simulink model "ServerExpCM_Model"  (R2023a)
settings: Solver=VariableStepAuto  StartTime=0.0  StopTime=10.0  RelTol=1e-3
libraries: NSA_DEVS_SINKS_ATOMIC x5, TimeSharedLib x4, NSA_DEVS_LOGISTICS_ATOMIC x2, NSA_DEVS_SOURCES_ATOMIC x1
settings Model: Creator=peter  LastModifiedBy=peter

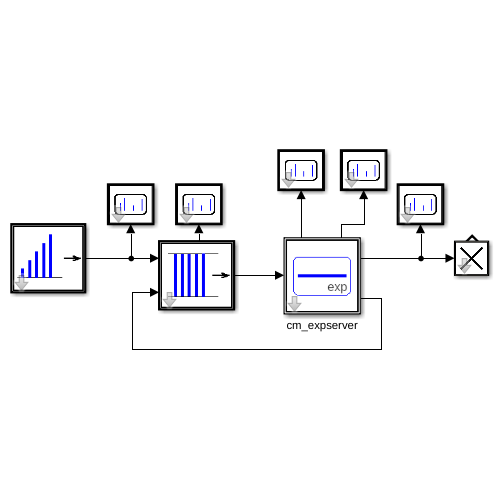
[thumbnail: Simulink's stored preview of the top-level diagram]
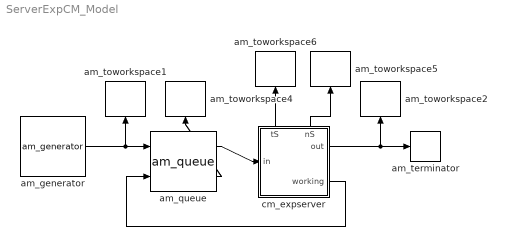
== system ServerExpCM_Model ==
  am_generator : NSA_DEVS_SOURCES_ATOMIC/am_generator  tG=1  n0=1  nG=10  tau=[0,1]  debug=0
      settings: SourceProductName=NSA_DEVS
  am_queue : NSA_DEVS_LOGISTICS_ATOMIC/am_queue  tD=[0,2]  tau=[0,1]  debug=0
      settings: SourceProductName=NSA_DEVS
  am_terminator : NSA_DEVS_LOGISTICS_ATOMIC/am_terminator  tau=[0,1]  debug=0
      settings: SourceProductName=NSA_DEVS
  am_toworkspace1 : NSA_DEVS_SINKS_ATOMIC/am_toworkspace  varname="\"genOut\""  t0=0  format="\"vector\""  tau=[0,3]  debug=0
      settings: SourceProductName=NSA_DEVS
  am_toworkspace2 : NSA_DEVS_SINKS_ATOMIC/am_toworkspace  varname="\"srvOut\""  t0=0  format="\"vector\""  tau=[0,3]  debug=0
      settings: SourceProductName=NSA_DEVS
  am_toworkspace4 : NSA_DEVS_SINKS_ATOMIC/am_toworkspace  varname="\"nqOut\""  t0=0  format="\"vector\""  tau=[0,3]  debug=0
      settings: SourceProductName=NSA_DEVS
  am_toworkspace5 : NSA_DEVS_SINKS_ATOMIC/am_toworkspace  varname="\"nsOut\""  t0=0  format="\"vector\""  tau=[0,5]  debug=0
      settings: SourceProductName=NSA_DEVS
  am_toworkspace6 : NSA_DEVS_SINKS_ATOMIC/am_toworkspace  varname="\"srvIn\""  t0=0  format="\"vector\""  tau=[0,3]  debug=0
      settings: SourceProductName=NSA_DEVS
  cm_expserver : Subsystem  mask{tS=0.9, tsField="serviceTime", tau=[0,1], debug=0}
      mask prompts: tS "mean service time"; tsField "field name for tS"
      settings: PortSchema="{\"entries\":[{\"content\":{\"sides\":[{\"content\":{\"connectorIds\":[\"In1\"]},\"type\":\"ConnectorPlacement.EquallySpacedRectSide\",\"uuid\":\"1bca0bff-f3fe-481b-89c0-36db42250c96\"},{\"content\":{\"connectorIds\":[\"Out1\",\"Out2\"],\"side\":\"RIGHT\"},\"type\":\"ConnectorPlacement.EquallySpacedRectSide\",\"uuid\":\"ba8183b4-e6da-42b8-a561-f6e51509f681\"},{\"content\":{\"connectorIds\":[\"Out3\",\"Out4\"],\"side\":\"TOP\"},\"type\":\"ConnectorPlacement.EquallySpacedRectSide\",\"uuid\":\"24a5b656-96e0-4e4a-b3a6-25d556caccb4\"}]},\"type\":\"ConnectorPlacement.EquallySpacedConnector\",\"uuid\":\"d4b4a1c8-ad66-47f2-a1d0-2811304b0058\"}],\"packageUris\":[\"http://schema.mathworks.com/mf0/Connector/R2020b\"],\"version\":\"1.0\"}"
      mask DialogControl Container4 Prompt: General
      mask DialogControl Container5 Prompt: Advanced
      mask Display: image('icon_expserver.png'); % Use "Edit Image" on toolstrip to change.
  wires:
  cm_expserver/4(nS) -> am_toworkspace5/1
  am_generator/1 -> am_queue/1, am_toworkspace1/1
  am_queue/2 -> am_toworkspace4/1
  cm_expserver/2(working) -> am_queue/2
  cm_expserver/3(tS) -> am_toworkspace6/1
  cm_expserver/1(out) -> am_toworkspace2/1, am_terminator/1
  am_queue/1 -> cm_expserver/1(in)

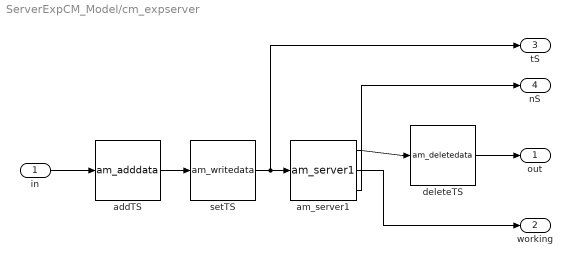
== system ServerExpCM_Model/cm_expserver ==
  in : Inport
  addTS : TimeSharedLib/am_adddata  fields=tsField  values="[\"1\"]"  numeric=[true]  infield="\"id\""  tau=0.25*tau  debug=debug
  am_server1 : TimeSharedLib/am_server1  tS=1.0  tsField=tsField  tau=0.5*tau  debug=debug
  deleteTS : TimeSharedLib/am_deletedata  fields=tsField  tau=0.25*tau  debug=debug
  setTS : TimeSharedLib/am_writedata  inFields=[]  outField=tsField  changeFunc="\"out = -\" + tS+ \"*log(rand());\""  tau=0.25*tau  debug=debug
  out : Outport
  working : Outport  Port=2
  tS : Outport  Port=3
  nS : Outport  Port=4
  wires:
  am_server1/1 -> deleteTS/1
  addTS/1 -> setTS/1
  deleteTS/1 -> out/1
  am_server1/2 -> working/1
  am_server1/3 -> nS/1
  setTS/1 -> tS/1, am_server1/1
  in/1 -> addTS/1
